simulink model "demodulateur_nc"  (R2021a)
settings: Solver=VariableStepAuto  StartTime=0.0  StopTime=10.0  RelTol=1e-3
libraries: dsparch4 x1
settings Model: Creator=jimmypan  LastModifiedBy=jimmypan

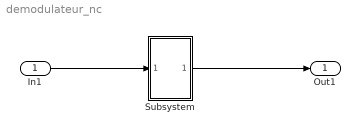
== system demodulateur_nc ==
  In1 : Inport
  Subsystem : Subsystem
  Out1 : Outport
  wires:
  In1/1 -> Subsystem/1(In1)
  Subsystem/1(Out1) -> Out1/1

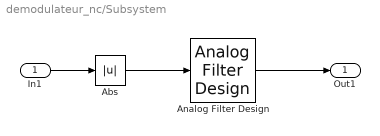
== system demodulateur_nc/Subsystem ==
  In1 : Inport
  Abs : Abs
  Analog Filter Design : dsparch4/Analog Filter Design  method=Butterworth  filttype=Lowpass  N=8  Wlo=130000  Whi=80  Rp=2  Rs=40
  Out1 : Outport
  wires:
  In1/1 -> Abs/1
  Analog Filter Design/1 -> Out1/1
  Abs/1 -> Analog Filter Design/1
